simulink model "Problem2"  (R2020b)
settings: Solver=VariableStepAuto  StartTime=0.0  StopTime=100  RelTol=1e-3
undefined symbols (not defined in the file): b, k1, k2, m1, m2
settings Model: Creator=omkar  LastModifiedBy=omkar

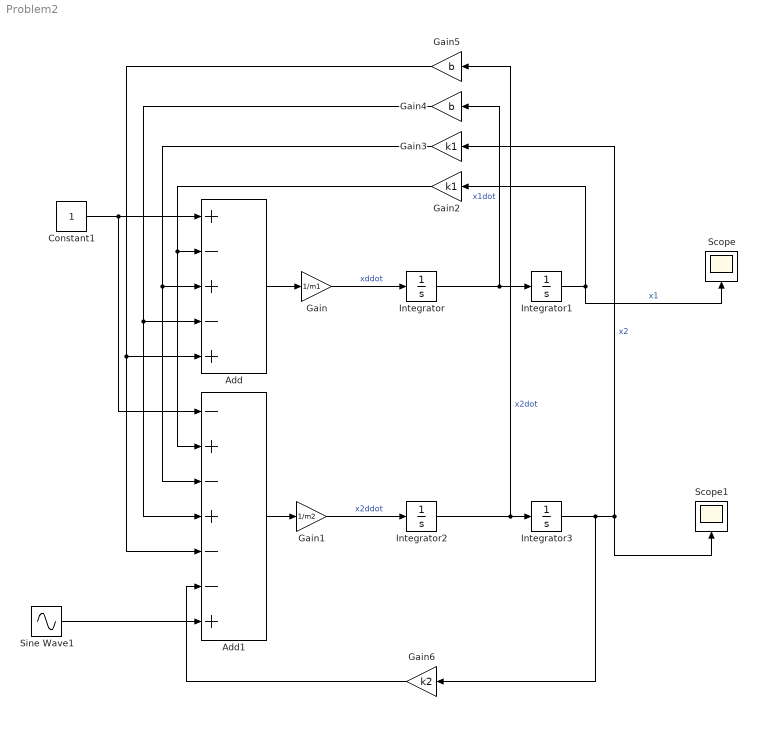
== system Problem2 ==
  Add : Sum  Inputs=+-+-+
  Add1 : Sum  Inputs=-+-+--+
  Constant1 : Constant
  Gain : Gain  Gain=1/m1
  Gain1 : Gain  Gain=1/m2
  Gain2 : Gain  Gain=k1
  Gain3 : Gain  Gain=k1
  Gain4 : Gain  Gain=b
  Gain5 : Gain  Gain=b
  Gain6 : Gain  Gain=k2
  Integrator{,1..3} (4 alike) : Integrator
  Scope : Scope
  Scope1 : Scope
  Sine Wave1 : Sin  Amplitude=k2  SampleTime=0
  wires:
  Sine Wave1/1 -> Add1/7
  Gain6/1 -> Add1/6
  Add1/1 -> Gain1/1
  Gain5/1 -> Add/5, Add1/5
  Gain4/1 -> Add/4, Add1/4
  Gain3/1 -> Add/3, Add1/3
  Gain2/1 -> Add/2, Add1/2
  Constant1/1 -> Add/1, Add1/1
  Add/1 -> Gain/1
  Integrator3/1 -> Scope1/1, Gain3/1, Gain6/1  "x2"
  Integrator2/1 -> Integrator3/1, Gain5/1  "x2dot"
  Gain1/1 -> Integrator2/1  "x2ddot"
  Integrator1/1 -> Gain2/1, Scope/1  "x1"
  Integrator/1 -> Integrator1/1, Gain4/1  "x1dot"
  Gain/1 -> Integrator/1  "xddot"
